simulink subsystem "Ground_Contact_Model"  (R2024b)
settings: Solver=VariableStepAuto  StartTime=0.0  StopTime=10.0  RelTol=1e-3
settings Model: Creator=thesa  LastModifiedBy=thesa

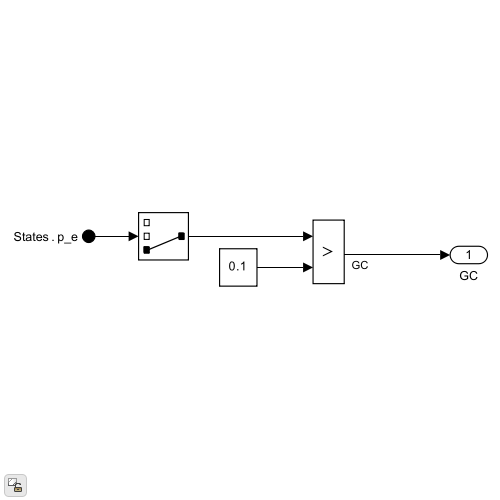
[thumbnail: Simulink's stored preview of the top-level diagram]
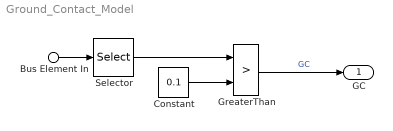
== system Ground_Contact_Model ==
  Bus Element In : Inport  PortName=States  Element=p_e
  Constant : Constant  Value=0.1
  GreaterThan : RelationalOperator  Operator=>  OutDataTypeStr=boolean  RndMeth=Simplest  InputSameDT=off
  Selector : Selector  InputPortWidth=3  IndexOptions=Index vector (dialog)  Indices=[3]  OutputSizes=1
  GC : Outport
  wires:
  Selector/1 -> GreaterThan/1
  GreaterThan/1 -> GC/1  "GC"
  Constant/1 -> GreaterThan/2
  Bus Element In/1 -> Selector/1
